simulink model "shiftregister1"  (R2025a)
settings: Solver=VariableStepAuto  StartTime=0.0  StopTime=10.0  RelTol=1e-3
libraries: StdLib x15
settings Model: Creator=peter  LastModifiedBy=peter
settings RTWCC: GPUComputeCapability=3.5

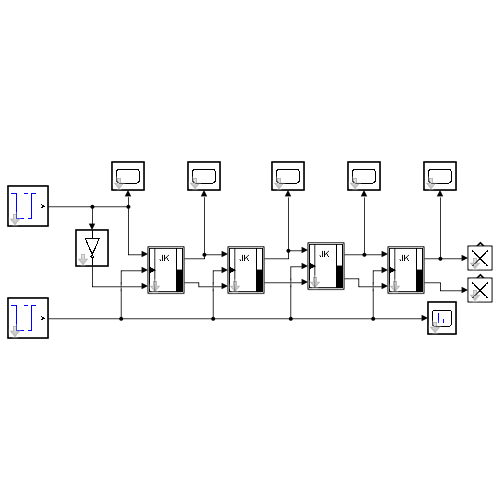
[thumbnail: Simulink's stored preview of the top-level diagram]
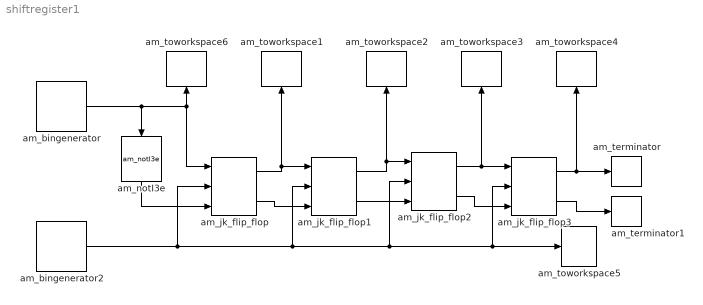
== system shiftregister1 ==
  am_bingenerator : StdLib/am_bingenerator  z0="\"0\""  tVec=[1, 2, 3, 4, 7, 9, 100]  tau=[0,1]  debug=0
  am_bingenerator2 : StdLib/am_bingenerator  z0="\"0\""  tVec=[0.5, 1.0]  tau=[0,1]  debug=0
  am_jk_flip_flop{,1..3} (4 alike) : StdLib/am_jk_flip_flop  q0="\"0\""  tau=[0,1]  debug=0
      settings: SourceProductName=FlipFlops
  am_notI3e : StdLib/am_notI3e  tau=[0,1]  debug=0
      settings: SourceProductName=Logic
  am_terminator : StdLib/am_terminator  tau=[0,1]  debug=0
  am_terminator1 : StdLib/am_terminator  tau=[0,1]  debug=0
  am_toworkspace1 : StdLib/am_toworkspace  varname="\"q1Out\""  t0=0  format="\"vector\""  tau=[0,5]  debug=0
  am_toworkspace2 : StdLib/am_toworkspace  varname="\"q2Out\""  t0=0  format="\"vector\""  tau=[0,5]  debug=0
  am_toworkspace3 : StdLib/am_toworkspace  varname="\"q3Out\""  t0=0  format="\"vector\""  tau=[0,5]  debug=0
  am_toworkspace4 : StdLib/am_toworkspace  varname="\"q4Out\""  t0=0  format="\"vector\""  tau=[0,5]  debug=0
  am_toworkspace5 : StdLib/am_toworkspace  varname="\"bin2Out\""  t0=0  format="\"vector\""  tau=[0,5]  debug=0
  am_toworkspace6 : StdLib/am_toworkspace  varname="\"bin1Out\""  t0=0  format="\"vector\""  tau=[0,5]  debug=0
  wires:
  am_jk_flip_flop/1 -> am_toworkspace1/1, am_jk_flip_flop1/1
  am_jk_flip_flop/2 -> am_jk_flip_flop1/3
  am_jk_flip_flop1/1 -> am_toworkspace2/1, am_jk_flip_flop2/1
  am_jk_flip_flop2/1 -> am_toworkspace3/1, am_jk_flip_flop3/1
  am_jk_flip_flop3/1 -> am_toworkspace4/1, am_terminator/1
  am_bingenerator/1 -> am_notI3e/1, am_toworkspace6/1, am_jk_flip_flop/1
  am_bingenerator2/1 -> am_jk_flip_flop/2, am_jk_flip_flop1/2, am_jk_flip_flop2/2, am_toworkspace5/1, am_jk_flip_flop3/2
  am_jk_flip_flop2/2 -> am_jk_flip_flop3/3
  am_jk_flip_flop3/2 -> am_terminator1/1
  am_notI3e/1 -> am_jk_flip_flop/3
  am_jk_flip_flop1/2 -> am_jk_flip_flop2/3
